simulink model "fw_pos_control"  (R2021a)
settings: Solver=FixedStepAuto  StartTime=0.0  StopTime=5  FixedStep=0.02  RelTol=1e-3
undefined symbols (not defined in the file): DiscIntNeverNeededParam, DT_DEFAULT, FW_AIRSPD_MAX, FW_AIRSPD_MIN, FW_L1_DAMPING, FW_L1_PERIOD, FW_L1_R_SLEW_MAX, FW_R_LIM, FW_T_CLMB_MAX, FW_T_HRATE_FF, FW_T_I_GAIN_PIT, FW_T_I_GAIN_THR, FW_T_PTCH_DAMP, FW_T_RLL2THR, FW_T_SEB_R_FF, FW_T_SINK_MAX, FW_T_SINK_MIN, FW_T_SPD_OMEGA, FW_T_STE_R_TC, FW_T_TAS_TC, FW_T_THR_DAMP, FW_T_VERT_ACC, FW_THR_CRUISE, FW_THR_MAX, FW_THR_MIN, FW_THR_SLEW_MAX, GRAVITY, magnitude
libraries: simulink x28, vrlib x3
(part 4 of 4)

== stateflow chart fw_pos_control/FW Control/fixed_wing.position_control.mode_action.tecs_controller/Tecs Logical ==
  state tecs_logical
    state detect_underspeed [parallel]
      en,du:
      TAS_min = tecs.eas_to_tas * TAS_min;
      TAS_max = tecs.eas_to_tas * TAS_max;
      % No underspeed protection in landing mode
      if ((tecs.mode == uint8(PX4_TECS_STATUS.TECS_MODE_LAND)) || ...
      (tecs.mode == uint8(PX4_TECS_STATUS.TECS_MODE_LAND_THROTTLELIM)))
      underspeed_detected = false;
      else
      underspeed_detected = true;
      end
      % 如果速度过小或者上次油门过大
      if (((tas < TAS_min * 0.9) && (last_throttle_setpoint >= tecs.throttle_max * 0.95)) || ...
      ((tecs.baro_altitude < tecs.hgt_setpoint) && underspeed_detected))
      underspeed_detected = true;
      else
      underspeed_detected = false;
      end
      settings: executionOrder=1
    state update_speed_height_weights [parallel]
      en,du:
      SKE_weighting_ = constrain(tecs.pitch_speed_weight, 0.0, 2.0);
      climbout_mode_active = tecs.climb_out_setpoint;
      if (underspeed_detected || climbout_mode_active)
      SKE_weighting_ = 2.0;
      end
      % don't allow any weight to be larger than one,
      % as it has the same effect as reducing the control
      % loop time constant and therefore can lead to a
      % destabilization of that control loop
      SPE_weighting_ = constrain(2.0 - SKE_weighting_, 0.0, 1.0);
      SKE_weighting_ = constrain(SKE_weighting_, 0.0, 1.0);
      settings: executionOrder=2
    state detect_uncommanded_descent [parallel]
      en,du:
      % If total energy is very low and reducing, throttle is high, and we are not in an
      % underspeed condition, then enter uncommanded descent recovery mode
      enter_mode = ~uncommanded_descent_recovery && ...
      ~underspeed_detected && (STE_error > 200.0) && ...
      (STE_rate < 0.0) && ...
      (last_throttle_setpoint >= tecs.throttle_max * 0.9);
      % If we enter an underspeed condition or recover the required total energy,
      % then exit uncommanded descent recovery mode
      exit_mode = uncommanded_descent_recovery && ...
      (underspeed_detected || (STE_error < 0.0));
      if (enter_mode)
      uncommanded_descent_recovery = true;
      elseif (exit_mode)
      uncommanded_descent_recovery = false;
      end
      settings: executionOrder=3
    state tecs_mode [parallel]
      en,du:
      % Set TECS mode for next frame
      if (underspeed_detected)
      tecs_mode = PX4_TECS_STATUS.TECS_MODE_UNDERSPEED;
      elseif (uncommanded_descent_recovery)
      tecs_mode = PX4_TECS_STATUS.TECS_MODE_BAD_DESCENT;
      elseif (tecs.climb_out_setpoint)
      tecs_mode = PX4_TECS_STATUS.TECS_MODE_CLIMBOUT;
      else
      % This is the default operation mode
      tecs_mode = PX4_TECS_STATUS.TECS_MODE_NORMAL;
      end
      settings: executionOrder=4
  data: TAS_min local single size=1; TAS_max local single size=1; climbout_mode_active local boolean size=1 =false; exit_mode local boolean size=1 =false; enter_mode local boolean; underspeed_detected output boolean size=1 =false; uncommanded_descent_recovery output boolean size=1 =false; SPE_weighting_ output single size=1 =single(1.0); SKE_weighting_ output single size=1 =single(1.0); tecs input Bus: px4_tecs_input; last_throttle_setpoint input single size=1; tas input single size=1; STE_rate input single size=1; STE_error input single size=1; tecs_mode output Enum: PX4_TECS_STATUS

== matlab function fw_pos_control/FW Control/fixed_wing.position_control.mode_action.l1_navigate_waypoints/MATLAB Function ==
  data: vector_A input; target_bearing output; vector_B input; vector_curr_position input; vector_AB_unit output; vector_A_to_airplane output; vector_B_to_P_unit output; ground_speed_vector input; ground_speed_3d output
% 主要计算L1算法中要使用到的向量,输出全部转为3维，方便后续使用叉乘
function [target_bearing, vector_AB_unit, vector_A_to_airplane, vector_B_to_P_unit, ground_speed_3d] = get_vector3d(vector_A, vector_B, vector_curr_position, ground_speed_vector)

% get the direction between the last (visited) and next waypoint
target_bearing = get_bearing_to_next_waypoint(vector_curr_position(1), vector_curr_position(2), vector_B(1), vector_B(2));

% calculate vector from A to B
vector_AB = get_local_planar_vector(vector_A, vector_B);

% check if waypoints are on top of each other. If yes,
% skip A and directly continue to B
% 如果上一个航点与当前航点距离很近，水平方向重合，高度不一样，飞机直接朝向当前航点
if (norm(vector_AB) < 1.0e-6)
    vector_AB = get_local_planar_vector(vector_curr_position, vector_B);
end

% 归一化
vector_AB_unit = [vector_AB / norm(vector_AB), single(0.0)];

% calculate the vector from waypoint A to the aircraft，上一个航点和飞机之间的向量
vector_A_to_airplane = [get_local_planar_vector(vector_A, vector_curr_position), single(0.0)];

% estimate airplane position WRT to B */
vector_B_to_P = get_local_planar_vector(vector_B, vector_curr_position);
vector_B_to_P_unit = [vector_B_to_P / norm(vector_B_to_P), single(0.0)];

% 地速转3维
ground_speed_3d = [ground_speed_vector, single(0.0)];

end
